simulink model "q_3dgyro_lqr"  (Simulink 7.8)
settings: Solver=ode2  StartTime=0.0  StopTime=inf  FixedStep=0.004  RelTol=1e-3
values from neighbouring files (symbols this model uses):
  A = [0 0 -h/Jy 0; 0 0 1 0; h/Jz 0 0 0; 0 1 0 0]    [setup_3dgyro.m]
  B = [1/Jy; 0; 0; 0]    [setup_3dgyro.m]
  CURRENT_LIMIT_MAX = 3    [setup_3dgyro.m]
  CURRENT_LIMIT_MIN = -CURRENT_LIMIT_MAX    (= -3)    [setup_3dgyro.m]
  DAC_LIMIT_MAX = 10    [setup_3dgyro.m]
  DAC_LIMIT_MIN = -DAC_LIMIT_MAX    (= -10)    [setup_3dgyro.m]
  K = lqr(A,B,Q,R)    [setup_3dgyro.m]
  K1 = lqr(A_w, B_w, Q_w, R_w)    [setup_3dgyro.m]
  Kt = 0.115    [setup_3dgyro.m]
  REFERENCE_RPM = 750    [setup_3dgyro.m]
undefined symbols (not defined in the file or in its folder): HIL, qc_get_step_size
libraries: simulink x8, quarc_library x6
settings Model: Creator=PKaram  LastModifiedBy=pmartin  SimulationMode=external  ExtModeTrigDuration=10000
settings SolverCC: PositivePriorityOrder=on
settings OptimizationCC: InitFltsAndDblsToZero=on
settings DebuggingCC: SaveWithParameterizedLinksMsg=none  MultiTaskDSMMsg=warning  MultiTaskCondExecSysMsg=none  FcnCallInpInsideContextMsg=Use local settings  StrictBusMsg=None
settings HardwareCC: TargetHWDeviceType=32-bit Generic
settings SFSimCC: SimParseCustomCode=off
settings RTWCC: SystemTargetFile=quarc_windows.tlc  TemplateMakefile=quarc_default_tmf  Description=QuaRC Win32 Target  ProcessScript=quarc_windows_make_rtw_hook  IncludeERTFirstTime=on
settings STFCustomTargetCC: TargetFcnLib=ansi_tfl_tmw.mat  TargetPreCompLibLocation=C:\PROGRA~2\QUARC\lib\2012b\windows\release  SystemTargetFile=quarc_windows.tlc
settings GRTTargetCC: TargetFcnLib=ansi_tfl_tmw.mat  TargetPreCompLibLocation=C:\PROGRA~2\QUARC\lib\2012b\windows\release  ParMdlRefBuildCompliant=off  CompOptLevelCompliant=off  ConcurrentExecutionCompliant=off  MatFileLogging=off  ExtMode=on  ExtModeMexFile=quarc_comm

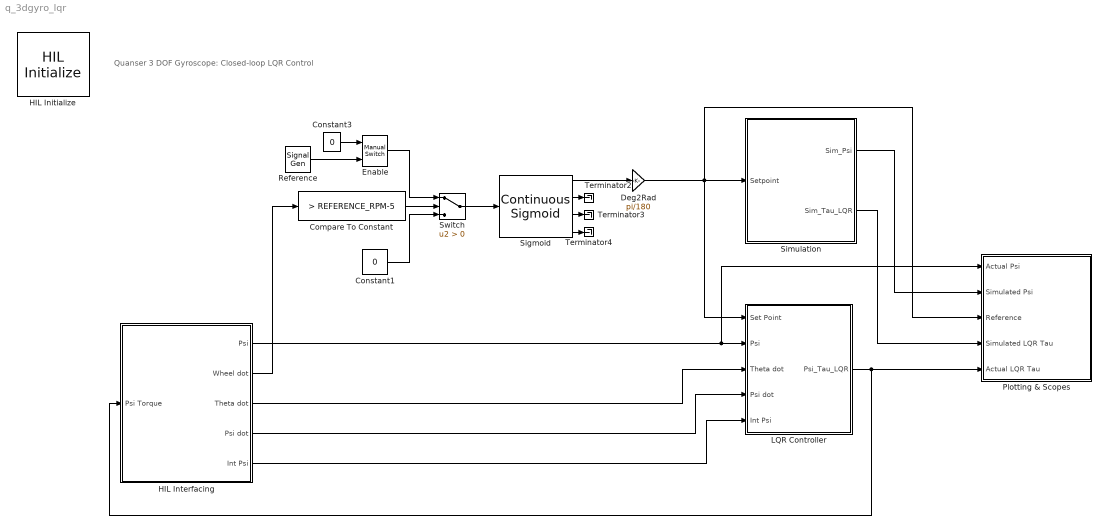
== system q_3dgyro_lqr ==
  note: Quanser 3 DOF Gyroscope:
      | Closed-loop LQR Control
  Compare To Constant : simulink/Logic and Bit Operations/Compare To Constant  relop=>  const=REFERENCE_RPM-5  OutDataTypeStr=uint8  ZeroCross=off
  Constant1 : Constant  Value=0
  Constant3 : Constant  Value=0
  Deg2Rad : Gain  Gain=pi/180
  Enable : simulink/Signal Routing/Manual Switch  sw=1  action=0  varsize=off
  HIL Initialize : quarc_library/Data Acquisition/Generic/Configuration/HIL Initialize  Priority=-99  object_name=HIL-1  board_type=q8_usb  board_number=0  board_options=update_rate=normal;decimation=1  exclusive=off  active=off  hardware_clocks=[0:2]  clock_modes=[]  initial_clock_frequencies=[]  set_clock_params_at_start=off  set_clock_params_at_switch_in=off  set_clock_frequencies_at_start=off  set_clock_frequencies_at_switch_in=off  analog_input_channels=[0:2]  analog_input_maximums=10  analog_input_minimums=-10  set_analog_input_params_at_start=on  set_analog_input_params_at_switch_in=off  analog_output_channels=[0:2]  analog_output_maximums=10  analog_output_minimums=-10  initial_analog_outputs=[0]  final_analog_outputs=[0]  watchdog_analog_outputs=0  set_analog_output_params_at_start=on  set_analog_output_params_at_switch_in=off  set_analog_outputs_at_start=on  set_analog_outputs_at_switch_in=off  set_analog_outputs_at_terminate=on  set_analog_outputs_at_switch_out=off  set_analog_outputs_on_watchdog=off  digital_input_channels=[]  digital_output_channels=[0:4]  digital_output_configuration=[]  initial_digital_outputs=[0 0 0 0 1]  final_digital_outputs=[1 1 1 1 0]  watchdog_digital_outputs=[1 1 1 1 0]  set_digital_output_params_at_start=off  set_digital_output_params_at_switch_in=off  set_digital_outputs_at_start=on  set_digital_outputs_at_switch_in=off  set_digital_outputs_at_terminate=on  set_digital_outputs_at_switch_out=off  set_digital_outputs_on_watchdog=off  encoder_channels=[0:7]  quadrature=[4]  encoder_filter_frequency=[]  initial_encoder_counts=[0]  set_encoder_params_at_start=on  set_encoder_params_at_switch_in=off  set_encoder_counts_at_start=on  set_encoder_counts_at_switch_in=off  pwm_channels=[0:7]  pwm_modes=0  pwm_frequency=99.532799999999995e6/4095  pwm_configuration=[0]  pwm_alignment=[0]  pwm_polarity=[1]  pwm_leading_deadband=[0]  pwm_trailing_deadband=[0]  initial_pwm_outputs=[0]  final_pwm_outputs=[0]  watchdog_pwm_outputs=[0]  set_pwm_params_at_start=on  set_pwm_params_at_switch_in=off  set_pwm_outputs_at_start=on  set_pwm_outputs_at_switch_in=off  set_pwm_outputs_at_terminate=on  set_pwm_outputs_at_switch_out=off  set_pwm_outputs_on_watchdog=off  other_output_channels=[]  initial_other_outputs=[]  final_other_outputs=[]  watchdog_other_outputs=[]  set_other_outputs_at_start=off  set_other_outputs_at_switch_in=off  set_other_outputs_at_terminate=off  set_other_outputs_at_switch_out=off  set_other_outputs_on_watchdog=off
  HIL Interfacing : Subsystem
  LQR Controller : Subsystem
  Plotting & Scopes : Subsystem
  Reference : SignalGenerator  WaveForm=square  Amplitude=20  Frequency=.1
  Sigmoid : quarc_library/Sources/Sigmoids/Continuous Sigmoid  params_source=Internal (dialog parameters)  max_velocity=SIGMOID_VEL_MAX  max_acceleration=SIGMOID_ACCEL_MAX  initial_position=0  initial_velocity=0  hold_off=0.5  input_sample_time=-1  output_sample_time=qc_get_step_size
  Simulation : Subsystem
  Switch : Switch  Criteria=u2 > Threshold
  Terminator2 : Terminator
  Terminator3 : Terminator
  Terminator4 : Terminator
  wires:
  HIL Interfacing/1(Psi) -> Plotting & Scopes/1(Actual Psi), LQR Controller/2(Psi)
  Simulation/1(Sim_Psi) -> Plotting & Scopes/2(Simulated Psi)
  LQR Controller/1(Psi_Tau_LQR) -> HIL Interfacing/1(Psi Torque), Plotting & Scopes/5(Actual LQR Tau)
  Sigmoid/1 -> Deg2Rad/1
  Compare To Constant/1 -> Switch/2
  Constant1/1 -> Switch/3
  Switch/1 -> Sigmoid/1
  Constant3/1 -> Enable/1
  Reference/1 -> Enable/2
  Enable/1 -> Switch/1
  Deg2Rad/1 -> LQR Controller/1(Set Point), Simulation/1(Setpoint), Plotting & Scopes/3(Reference)
  Sigmoid/2 -> Terminator2/1
  Sigmoid/3 -> Terminator3/1
  Sigmoid/4 -> Terminator4/1
  HIL Interfacing/5(Int Psi) -> LQR Controller/5(Int Psi)
  HIL Interfacing/3(Theta dot) -> LQR Controller/3(Theta dot)
  HIL Interfacing/4(Psi dot) -> LQR Controller/4(Psi dot)
  Simulation/2(Sim_Tau_LQR) -> Plotting & Scopes/4(Simulated LQR Tau)
  HIL Interfacing/2(Wheel dot) -> Compare To Constant/1

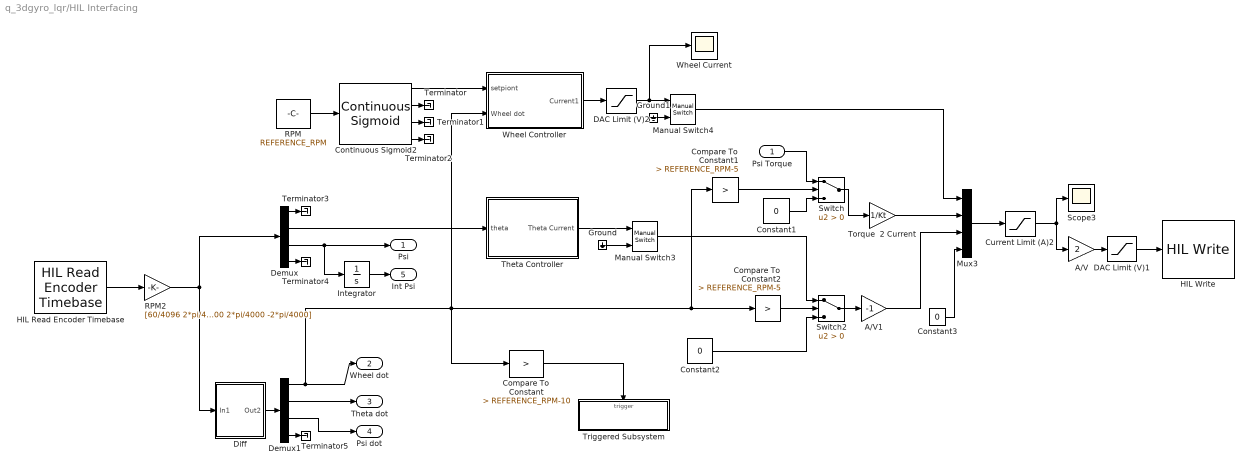
== system q_3dgyro_lqr/HIL Interfacing ==
  Psi Torque : Inport
  A/V : Gain  Gain=2
  A/V1 : Gain  Gain=-1
  Compare To Constant : simulink/Logic and Bit Operations/Compare To Constant  relop=>  const=REFERENCE_RPM-10  OutDataTypeStr=uint8  ZeroCross=off
  Compare To Constant1 : simulink/Logic and Bit Operations/Compare To Constant  relop=>  const=REFERENCE_RPM-5  OutDataTypeStr=uint8  ZeroCross=off
  Compare To Constant2 : simulink/Logic and Bit Operations/Compare To Constant  relop=>  const=REFERENCE_RPM-5  OutDataTypeStr=uint8  ZeroCross=off
  Constant1 : Constant  Value=0
  Constant2 : Constant  Value=0
  Constant3 : Constant  Value=0
  Continuous Sigmoid2 : quarc_library/Sources/Sigmoids/Continuous Sigmoid  params_source=Internal (dialog parameters)  max_velocity=250  max_acceleration=250  initial_position=0  initial_velocity=0  hold_off=0.5  input_sample_time=-1  output_sample_time=qc_get_step_size
  Current Limit (A)2 : Saturate  UpperLimit=CURRENT_LIMIT_MAX  LowerLimit=CURRENT_LIMIT_MIN
  DAC Limit (V)1 : Saturate  UpperLimit=DAC_LIMIT_MAX  LowerLimit=DAC_LIMIT_MIN
  DAC Limit (V)2 : Saturate  UpperLimit=1  LowerLimit=-1
  Demux : Demux
  Demux1 : Demux
  Diff : Subsystem
  Ground : Ground
  Ground1 : Ground
  HIL Read Encoder Timebase : quarc_library/Data Acquisition/Generic/Timebases/HIL Read Encoder Timebase  object_name=HIL-1  clock=0  channels=0:3  samples_in_buffer=max(ceil(1/qc_get_step_size), 1)  active=on  vector_output=on  data_type_mode=Inherit via back propagation  data_type=double
  HIL Write : quarc_library/Data Acquisition/Generic/Immediate I//O/HIL Write  object_name=HIL-1  analog_channels=0:3  pwm_channels=[]  digital_channels=[]  other_channels=[]  sample_time=-1  active=off  vector_input=on
  Integrator : Integrator
  Manual Switch3 : simulink/Signal Routing/Manual Switch  sw=1  action=0  varsize=off
  Manual Switch4 : simulink/Signal Routing/Manual Switch  sw=1  action=0  varsize=off
  Mux3 : Mux
  RPM : Constant  Value=REFERENCE_RPM
  RPM2 : Gain  Gain=[60/4096 2*pi/4000 2*pi/4000 -2*pi/4000]
  Scope3 : Scope
      settings: TimeRange=10  YMin=-3.5  YMax=3.5  SaveName=ScopeData7
  Switch : Switch  Criteria=u2 > Threshold
  Switch2 : Switch  Criteria=u2 > Threshold
  Terminator{,1..5} (6 alike) : Terminator
  Theta Controller : Subsystem
  Torque  2 Current : Gain  Gain=1/Kt
  Triggered Subsystem : Subsystem  TreatAsAtomicUnit=on
  Wheel Controller : Subsystem
  Wheel Current : Scope
      settings: YMin=-0.2  YMax=0.55  SaveName=ScopeData3
  Psi : Outport
  Wheel dot : Outport  Port=2
  Theta dot : Outport  Port=3
  Psi dot : Outport  Port=4
  Int Psi : Outport  Port=5
  wires:
  HIL Read Encoder Timebase/1 -> RPM2/1
  RPM2/1 -> Demux/1, Diff/1(In1)
  Diff/1(Out2) -> Demux1/1
  Demux1/2 -> Theta dot/1
  A/V/1 -> DAC Limit (V)1/1
  DAC Limit (V)1/1 -> HIL Write/1
  Demux/2 -> Theta Controller/1(theta)
  Theta Controller/1(Theta Current) -> Manual Switch3/1
  RPM/1 -> Continuous Sigmoid2/1
  Continuous Sigmoid2/1 -> Wheel Controller/1(setpiont)
  DAC Limit (V)2/1 -> Manual Switch4/1, Wheel Current/1
  Current Limit (A)2/1 -> A/V/1, Scope3/1
  Demux1/1 -> Wheel Controller/2(Wheel dot), Compare To Constant/1, Compare To Constant2/1, Compare To Constant1/1, Wheel dot/1
  Psi Torque/1 -> Switch/1
  Constant1/1 -> Switch/3
  Switch/1 -> Torque  2 Current/1
  Compare To Constant1/1 -> Switch/2
  Manual Switch3/1 -> Switch2/1
  Compare To Constant2/1 -> Switch2/2
  Constant2/1 -> Switch2/3
  Switch2/1 -> A/V1/1
  Wheel Controller/1(Current1) -> DAC Limit (V)2/1
  Integrator/1 -> Int Psi/1
  Torque  2 Current/1 -> Mux3/2
  Manual Switch4/1 -> Mux3/1
  Mux3/1 -> Current Limit (A)2/1
  Demux/3 -> Integrator/1, Psi/1
  Demux1/3 -> Psi dot/1
  A/V1/1 -> Mux3/3
  Constant3/1 -> Mux3/4
  Compare To Constant/1 -> Triggered Subsystem/Trigger
  Continuous Sigmoid2/2 -> Terminator/1
  Continuous Sigmoid2/3 -> Terminator1/1
  Continuous Sigmoid2/4 -> Terminator2/1
  Ground1/1 -> Manual Switch4/2
  Ground/1 -> Manual Switch3/2
  Demux/1 -> Terminator3/1
  Demux/4 -> Terminator4/1
  Demux1/4 -> Terminator5/1

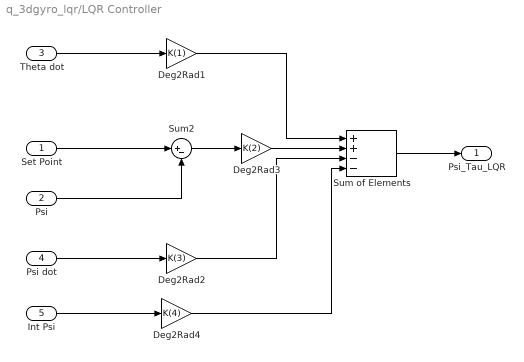
== system q_3dgyro_lqr/LQR Controller ==
  Set Point : Inport
  Psi : Inport  Port=2
  Theta dot : Inport  Port=3
  Psi dot : Inport  Port=4
  Int Psi : Inport  Port=5
  Deg2Rad1 : Gain  Gain=K(1)
  Deg2Rad2 : Gain  Gain=K(3)
  Deg2Rad3 : Gain  Gain=K(2)
  Deg2Rad4 : Gain  Gain=K(4)
  Sum of Elements : Sum  Inputs=++--
  Sum2 : Sum  Inputs=|+-
  Psi_Tau_LQR : Outport
  wires:
  Set Point/1 -> Sum2/1
  Psi/1 -> Sum2/2
  Sum2/1 -> Deg2Rad3/1
  Sum of Elements/1 -> Psi_Tau_LQR/1
  Deg2Rad1/1 -> Sum of Elements/1
  Deg2Rad3/1 -> Sum of Elements/2
  Deg2Rad2/1 -> Sum of Elements/3
  Int Psi/1 -> Deg2Rad4/1
  Deg2Rad4/1 -> Sum of Elements/4
  Theta dot/1 -> Deg2Rad1/1
  Psi dot/1 -> Deg2Rad2/1

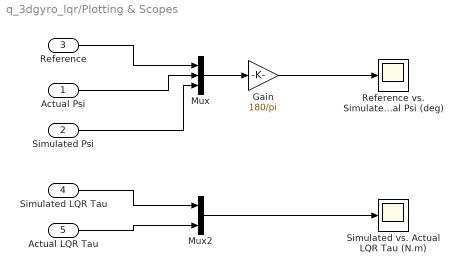
== system q_3dgyro_lqr/Plotting & Scopes ==
  Actual Psi : Inport
  Simulated Psi : Inport  Port=2
  Reference : Inport  Port=3
  Simulated LQR Tau : Inport  Port=4
  Actual LQR Tau : Inport  Port=5
  Gain : Gain  Gain=180/pi
  Mux : Mux  Inputs=3
  Mux2 : Mux  Inputs=2
  Reference vs. Simulated vs. Actual Psi (deg) : Scope
      settings: TimeRange=10  YMin=-30  YMax=30  SaveName=rsp_psi
  Simulated vs. Actual LQR Tau (N.m) : Scope
      settings: YMin=-2  YMax=2  SaveName=rsp_tau
  wires:
  Reference/1 -> Mux/1
  Actual Psi/1 -> Mux/2
  Simulated Psi/1 -> Mux/3
  Mux/1 -> Gain/1
  Simulated LQR Tau/1 -> Mux2/1
  Actual LQR Tau/1 -> Mux2/2
  Mux2/1 -> Simulated vs. Actual LQR Tau (N.m)/1
  Gain/1 -> Reference vs. Simulated vs. Actual Psi (deg)/1

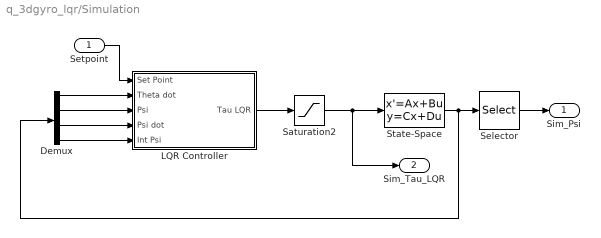
== system q_3dgyro_lqr/Simulation ==
  Setpoint : Inport
  Demux : Demux
  LQR Controller : Subsystem
  Saturation2 : Saturate  UpperLimit=1.5  LowerLimit=-1.5
  Selector : Selector  InputPortWidth=4  IndexOptions=Index vector (dialog)  Indices=2  OutputSizes=1
  State-Space : StateSpace  A=A  B=B  C=eye(4)  D=zeros(4,1)  X0=[0 0 0 0]
  Sim_Psi : Outport
  Sim_Tau_LQR : Outport  Port=2
  wires:
  LQR Controller/1(Tau LQR) -> Saturation2/1
  Saturation2/1 -> Sim_Tau_LQR/1, State-Space/1
  Setpoint/1 -> LQR Controller/1(Set Point)
  Demux/1 -> LQR Controller/2(Theta dot)
  Demux/2 -> LQR Controller/3(Psi)
  Demux/3 -> LQR Controller/4(Psi dot)
  Demux/4 -> LQR Controller/5(Int Psi)
  State-Space/1 -> Selector/1, Demux/1
  Selector/1 -> Sim_Psi/1

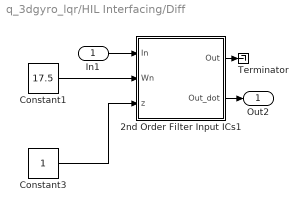
== system q_3dgyro_lqr/HIL Interfacing/Diff ==
  In1 : Inport
  2nd Order Filter Input ICs1 : Subsystem
  Constant1 : Constant  Value=17.5
  Constant3 : Constant
  Terminator : Terminator
  Out2 : Outport
  wires:
  Constant1/1 -> 2nd Order Filter Input ICs1/2(Wn)
  Constant3/1 -> 2nd Order Filter Input ICs1/3(z)
  In1/1 -> 2nd Order Filter Input ICs1/1(In)
  2nd Order Filter Input ICs1/2(Out_dot) -> Out2/1
  2nd Order Filter Input ICs1/1(Out) -> Terminator/1

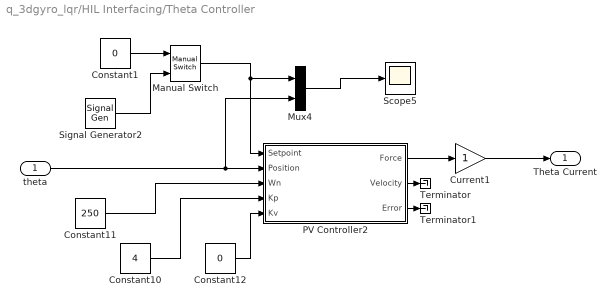
== system q_3dgyro_lqr/HIL Interfacing/Theta Controller ==
  theta : Inport
  Constant1 : Constant  Value=0
  Constant10 : Constant  Value=4
  Constant11 : Constant  Value=250
  Constant12 : Constant  Value=0
  Current1 : Gain
  Manual Switch : simulink/Signal Routing/Manual Switch  sw=1  action=0  varsize=off
  Mux4 : Mux  Inputs=2
  PV Controller2 : Subsystem
  Scope5 : Scope
      settings: TimeRange=10  YMin=-0.4  YMax=0.3  SaveName=ScopeData6
  Signal Generator2 : SignalGenerator  WaveForm=square  Amplitude=0  Frequency=.1
  Terminator : Terminator
  Terminator1 : Terminator
  Theta Current : Outport
  wires:
  theta/1 -> Mux4/2, PV Controller2/2(Position)
  Constant11/1 -> PV Controller2/3(Wn)
  Constant10/1 -> PV Controller2/4(Kp)
  Constant12/1 -> PV Controller2/5(Kv)
  PV Controller2/1(Force) -> Current1/1
  Mux4/1 -> Scope5/1
  Current1/1 -> Theta Current/1
  Signal Generator2/1 -> Manual Switch/2
  Constant1/1 -> Manual Switch/1
  Manual Switch/1 -> PV Controller2/1(Setpoint), Mux4/1
  PV Controller2/2(Velocity) -> Terminator/1
  PV Controller2/3(Error) -> Terminator1/1

== system q_3dgyro_lqr/HIL Interfacing/Triggered Subsystem ==
  Trigger : TriggerPort
  HIL Set Encoder Counts : quarc_library/Data Acquisition/Generic/Configuration/HIL Set Encoder Counts  object_name=HIL-1  channels=2  source=internal  counts=0  sample_time=-1  active=on  vector_input=on
      settings: AttributesFormatString=(%<object_name>)

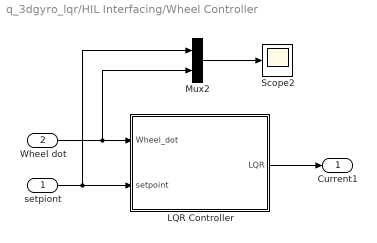
== system q_3dgyro_lqr/HIL Interfacing/Wheel Controller ==
  setpiont : Inport
  Wheel dot : Inport  Port=2
  LQR Controller : Subsystem
  Mux2 : Mux  Inputs=2
  Scope2 : Scope
      settings: YMin=699.2  YMax=700.6  SaveName=ScopeData2
  Current1 : Outport
  wires:
  LQR Controller/1(LQR) -> Current1/1
  setpiont/1 -> LQR Controller/2(setpoint), Mux2/1
  Wheel dot/1 -> LQR Controller/1(Wheel_dot), Mux2/2
  Mux2/1 -> Scope2/1

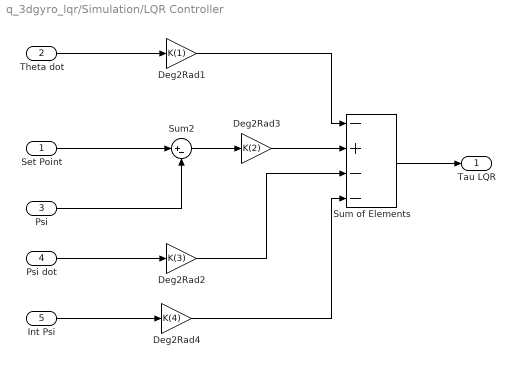
== system q_3dgyro_lqr/Simulation/LQR Controller ==
  Set Point : Inport
  Theta dot : Inport  Port=2
  Psi : Inport  Port=3
  Psi dot : Inport  Port=4
  Int Psi : Inport  Port=5
  Deg2Rad1 : Gain  Gain=K(1)
  Deg2Rad2 : Gain  Gain=K(3)
  Deg2Rad3 : Gain  Gain=K(2)
  Deg2Rad4 : Gain  Gain=K(4)
  Sum of Elements : Sum  Inputs=-+--
  Sum2 : Sum  Inputs=|+-
  Tau LQR : Outport
  wires:
  Sum2/1 -> Deg2Rad3/1
  Sum of Elements/1 -> Tau LQR/1
  Deg2Rad1/1 -> Sum of Elements/1
  Deg2Rad3/1 -> Sum of Elements/2
  Int Psi/1 -> Deg2Rad4/1
  Deg2Rad2/1 -> Sum of Elements/3
  Deg2Rad4/1 -> Sum of Elements/4
  Set Point/1 -> Sum2/1
  Theta dot/1 -> Deg2Rad1/1
  Psi/1 -> Sum2/2
  Psi dot/1 -> Deg2Rad2/1

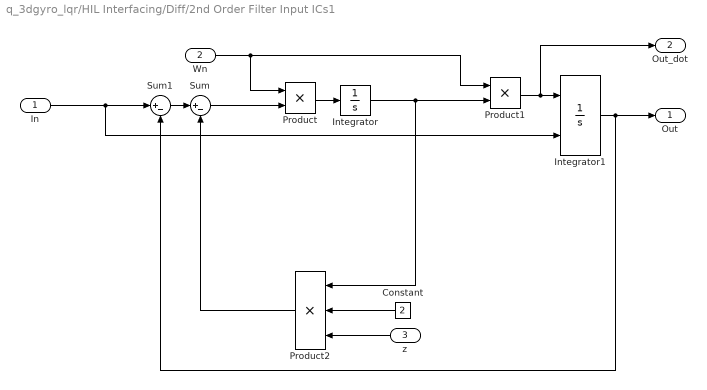
== system q_3dgyro_lqr/HIL Interfacing/Diff/2nd Order Filter Input ICs1 ==
  In : Inport
  Wn : Inport  Port=2
  z : Inport  Port=3
  Constant : Constant  Value=2
  Integrator : Integrator
  Integrator1 : Integrator  InitialConditionSource=external
  Product : Product  RndMeth=Zero
  Product1 : Product  RndMeth=Zero
  Product2 : Product  Inputs=3  RndMeth=Zero
  Sum : Sum  Inputs=|+-
  Sum1 : Sum  Inputs=|+-
  Out : Outport
  Out_dot : Outport  Port=2
  wires:
  Constant/1 -> Product2/2
  z/1 -> Product2/3
  Product2/1 -> Sum/2
  In/1 -> Integrator1/2, Sum1/1
  Sum1/1 -> Sum/1
  Integrator1/1 -> Out/1, Sum1/2
  Integrator/1 -> Product2/1, Product1/2
  Product1/1 -> Out_dot/1, Integrator1/1
  Wn/1 -> Product1/1, Product/1
  Sum/1 -> Product/2
  Product/1 -> Integrator/1

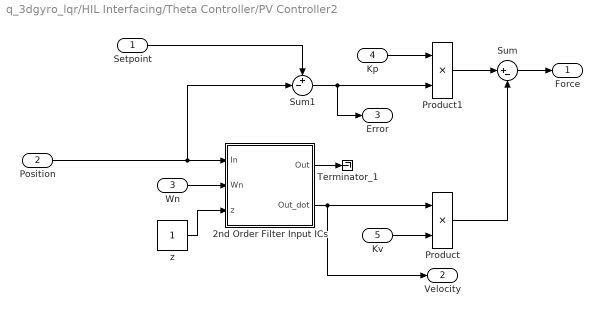
== system q_3dgyro_lqr/HIL Interfacing/Theta Controller/PV Controller2 ==
  Setpoint : Inport
  Position : Inport  Port=2
  Wn : Inport  Port=3
  Kp : Inport  Port=4
  Kv : Inport  Port=5
  2nd Order Filter Input ICs : Subsystem
  Product : Product  RndMeth=Zero
  Product1 : Product  RndMeth=Zero
  Sum : Sum  Inputs=|+-
  Sum1 : Sum  Inputs=+-|
  Terminator_1 : Terminator
  z : Constant
  Force : Outport
  Velocity : Outport  Port=2
  Error : Outport  Port=3
  wires:
  Wn/1 -> 2nd Order Filter Input ICs/2(Wn)
  z/1 -> 2nd Order Filter Input ICs/3(z)
  Position/1 -> 2nd Order Filter Input ICs/1(In), Sum1/2
  2nd Order Filter Input ICs/2(Out_dot) -> Velocity/1, Product/1
  Kp/1 -> Product1/1
  Setpoint/1 -> Sum1/1
  Sum1/1 -> Product1/2, Error/1
  Product1/1 -> Sum/1
  Kv/1 -> Product/2
  Product/1 -> Sum/2
  Sum/1 -> Force/1
  2nd Order Filter Input ICs/1(Out) -> Terminator_1/1

== system q_3dgyro_lqr/HIL Interfacing/Wheel Controller/LQR Controller ==
  Wheel_dot : Inport
  setpoint : Inport  Port=2
  Gain1 : Gain  Gain=K1
  Sum : Sum  Inputs=|+-
  LQR : Outport
  wires:
  Gain1/1 -> LQR/1
  setpoint/1 -> Sum/1
  Wheel_dot/1 -> Sum/2
  Sum/1 -> Gain1/1

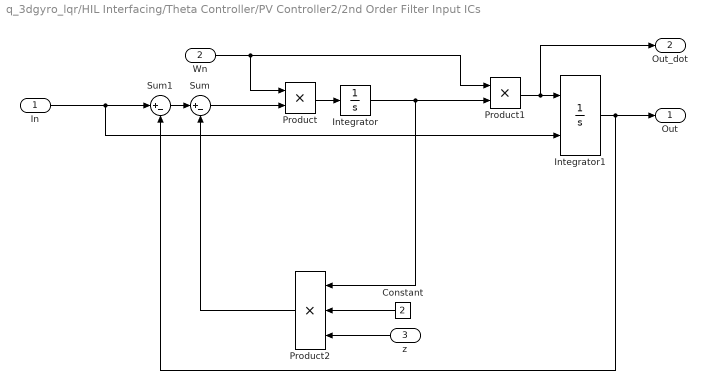
== system q_3dgyro_lqr/HIL Interfacing/Theta Controller/PV Controller2/2nd Order Filter Input ICs ==
  In : Inport
  Wn : Inport  Port=2
  z : Inport  Port=3
  Constant : Constant  Value=2
  Integrator : Integrator
  Integrator1 : Integrator  InitialConditionSource=external
  Product : Product  RndMeth=Zero
  Product1 : Product  RndMeth=Zero
  Product2 : Product  Inputs=3  RndMeth=Zero
  Sum : Sum  Inputs=|+-
  Sum1 : Sum  Inputs=|+-
  Out : Outport
  Out_dot : Outport  Port=2
  wires:
  Constant/1 -> Product2/2
  z/1 -> Product2/3
  Product2/1 -> Sum/2
  In/1 -> Integrator1/2, Sum1/1
  Sum1/1 -> Sum/1
  Integrator1/1 -> Out/1, Sum1/2
  Integrator/1 -> Product2/1, Product1/2
  Product1/1 -> Out_dot/1, Integrator1/1
  Wn/1 -> Product1/1, Product/1
  Sum/1 -> Product/2
  Product/1 -> Integrator/1
